simulink model "AverageTemp"  (R2023b)
settings: Solver=VariableStepAuto  StartTime=0.0  StopTime=10.0  RelTol=1e-3
settings Model: Creator=ant  LastModifiedBy=ant

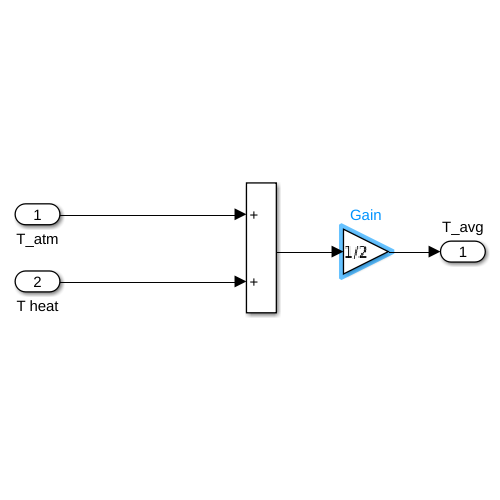
[thumbnail: Simulink's stored preview of the top-level diagram]
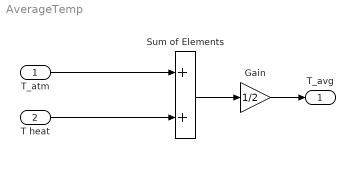
== system AverageTemp ==
  T_atm : Inport
  T heat : Inport  Port=2
  Gain : Gain  Gain=1/2
  Sum of Elements : Sum
  T_avg : Outport  VectorParamsAs1DForOutWhenUnconnected=off
  wires:
  T_atm/1 -> Sum of Elements/1
  T heat/1 -> Sum of Elements/2
  Gain/1 -> T_avg/1
  Sum of Elements/1 -> Gain/1
